simulink model "SPIcontroller"  (R2014b)
settings: Solver=FixedStepDiscrete  StartTime=0.0  StopTime=inf  FixedStep=1  RelTol=1e-3
undefined symbols (not defined in the file): PROD_ID
libraries: hdlsllib x1, simulink x1
settings Model: Creator=bsoheili  LastModifiedBy=dlwalter
settings DataIOCC: SaveOutput=off  SaveTime=off
settings OptimizationCC: BlockReduction=off  ConditionallyExecuteInputs=off  InlineParams=on  UseDivisionForNetSlopeComputation=UseDivisionForReciprocalsOfIntegersOnly  UseFloatMulNetSlope=on  InlineInvariantSignals=on  EnhancedBackFolding=on  EfficientFloat2IntCast=on  OptimizeModelRefInitCode=on  LifeSpan=1
settings DebuggingCC: AlgebraicLoopMsg=error  InheritedTsInSrcMsg=none  StrictBusMsg=ErrorOnBusTreatedAsVector  NonBusSignalsTreatedAsBus=error
settings HardwareCC: ProdHWDeviceType=ASIC/FPGA->ASIC/FPGA  ProdEqTarget=off
settings RTWCC: SystemTargetFile=ert.tlc  TemplateMakefile=ert_default_tmf  Description=Embedded Coder  GenerateReport=on  ProcessScript=ert_make_rtw_hook  IncludeHyperlinkInReport=on  LaunchReport=on  GenerateTraceInfo=on  GenerateTraceReport=on  GenerateTraceReportSl=on  GenerateTraceReportSf=on  GenerateTraceReportEml=on  GenerateCodeMetricsReport=on
settings CodeAppCC: IgnoreCustomStorageClasses=off
settings ERTTargetCC: GenerateSampleERTMain=on  CombineSignalStateStructs=on  SuppressErrorStatus=on  InlinedParameterPlacement=NonHierarchical  ERTCustomFileTemplate=example_file_process.tlc

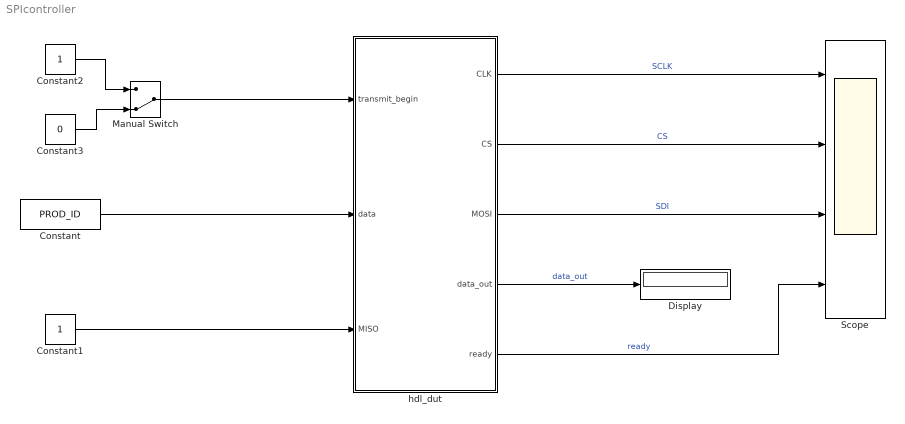
== system SPIcontroller ==
  Constant : Constant  Value=PROD_ID  OutDataTypeStr=fixdt(0,16,0)  SampleTime=-1
  Constant1 : Constant  OutDataTypeStr=boolean  SampleTime=-1
  Constant2 : Constant  OutDataTypeStr=boolean  SampleTime=-1
  Constant3 : Constant  Value=0  OutDataTypeStr=boolean  SampleTime=-1
  Display : Display
  Manual Switch : ManualSwitch  CurrentSetting=0
  Scope : Scope  NumInputPorts=4
      settings: YMin=-2~-2~-2~-5  YMax=2~2~2~5
  hdl_dut : Subsystem  TreatAsAtomicUnit=on  mask{message_length=16, clk_freq=1e6, cs_to_clk_edge=40, stall_time=2}
      mask DialogControl Control2 Prompt: SPI Controller Parameters
      mask DialogControl Control6 Prompt: Message Length (bits)
      mask DialogControl Control3 Prompt: Clock Frequency
      mask DialogControl Control4 Prompt: Chip Select to Clock edge Time (ns)
      mask DialogControl Control5 Prompt: Stall Time (us)
  wires:
  Constant/1 -> hdl_dut/2(data)
  Constant2/1 -> Manual Switch/1
  Constant3/1 -> Manual Switch/2
  Manual Switch/1 -> hdl_dut/1(transmit_begin)
  Constant1/1 -> hdl_dut/3(MISO)
  hdl_dut/1(CLK) -> Scope/1  "SCLK"
  hdl_dut/2(CS) -> Scope/2  "CS"
  hdl_dut/3(MOSI) -> Scope/3  "SDI"
  hdl_dut/4(data_out) -> Display/1  "data_out"
  hdl_dut/5(ready) -> Scope/4  "ready"

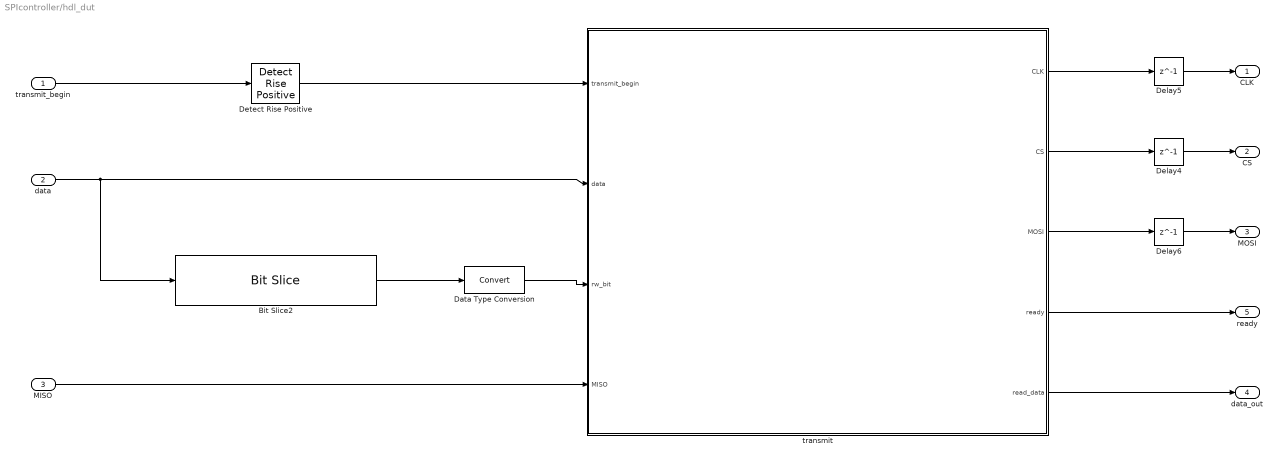
== system SPIcontroller/hdl_dut ==
  transmit_begin : Inport
  data : Inport  Port=2
  MISO : Inport  Port=3
  Bit Slice2 : hdlsllib/HDL Operations/Bit Slice  lidx=message_length-1  ridx=message_length-1
  Data Type Conversion : DataTypeConversion
  Delay4 : Delay  DelayLength=1  InitialCondition=1
  Delay5 : Delay  DelayLength=1  InitialCondition=1
  Delay6 : Delay  DelayLength=1  InitialCondition=0
  Detect Rise Positive : simulink/Logic and Bit Operations/Detect Rise Positive  vinit=0  InputProcessing=Inherited  OutDataTypeStr=boolean
  transmit : Stateflow chart  TreatAsAtomicUnit=on
  CLK : Outport
  CS : Outport  Port=2
  MOSI : Outport  Port=3
  data_out : Outport  Port=4
  ready : Outport  Port=5
  wires:
  data/1 -> Bit Slice2/1, transmit/2(data)
  Delay4/1 -> CS/1
  Delay5/1 -> CLK/1
  Delay6/1 -> MOSI/1
  Bit Slice2/1 -> Data Type Conversion/1
  transmit_begin/1 -> Detect Rise Positive/1
  Data Type Conversion/1 -> transmit/3(rw_bit)
  MISO/1 -> transmit/4(MISO)
  Detect Rise Positive/1 -> transmit/1(transmit_begin)
  transmit/2(CS) -> Delay4/1
  transmit/1(CLK) -> Delay5/1
  transmit/3(MOSI) -> Delay6/1
  transmit/5(read_data) -> data_out/1
  transmit/4(ready) -> ready/1

== stateflow chart SPIcontroller/hdl_dut/transmit ==
  settings: executeAtInitialization=1
  state IDLE
  state BEGIN
  state CHIPSELECT
  state WRITE
    state CLOCK_BEGIN
    state CLOCK_HIGH
    state CLOCK_LOW
    state CLOCK_END
    (default) -> CLOCK_BEGIN
    CLOCK_BEGIN -> CLOCK_LOW : {CLK = false;
        | bit_count = 0;}
    CLOCK_LOW -> CLOCK_HIGH [order 1] : [count == clk_wait]
        | {CLK = 1; count = 0;bit_count ++;
        | MOSI = sdi_gen(data, bit_count);}
    CLOCK_HIGH -> CLOCK_HIGH [order 3] : {count++;}
    CLOCK_LOW -> CLOCK_LOW [order 2] : {count++;}
    CLOCK_HIGH -> CLOCK_LOW [order 1] : [count == clk_wait]
        | {CLK = 0; count = 0;}
    CLOCK_HIGH -> CLOCK_END [order 2] : [bit_count == message_length]
        | {count = 0; transmit_flag = 0; MOSI = 0;}
  state READ
    state CLOCK_BEGIN1
    state BEGIN_READ
    state CLOCK_HIGH1
    state CLOCK_LOW1
    state CS_LOW
    state CLOCK_BEGIN2
    state CLOCK_END1
    state STALL1
    state CLOCK_HIGH2
    state CLOCK_LOW2
    state CLOCK_END2
    (default) -> CLOCK_BEGIN1
    CLOCK_BEGIN1 -> CLOCK_LOW1 : {CLK = false;
        | bit_count = 0;}
    STALL1 -> BEGIN_READ [order 1] : [count == stall_wait]
        | {count = 0;}
    BEGIN_READ -> BEGIN_READ [order 2] : {count++;}
    CLOCK_LOW1 -> CLOCK_HIGH1 [order 1] : [count == clk_wait]
        | {CLK = 1; count = 0;bit_count ++;
        | MOSI = sdi_gen(data, bit_count);}
    CLOCK_HIGH1 -> CLOCK_HIGH1 [order 3] : {count++;}
    CLOCK_LOW1 -> CLOCK_LOW1 [order 2] : {count++;}
    BEGIN_READ -> CS_LOW [order 1] : [count == 10]{CS = 0;count = 0;}
    CLOCK_HIGH1 -> CLOCK_LOW1 [order 1] : [count == clk_wait]
        | {CLK = 0; count = 0;}
    CLOCK_HIGH1 -> CLOCK_END1 [order 2] : [bit_count == message_length]
        | {count = 0; MOSI = 0;}
    CS_LOW -> CS_LOW [order 2] : {count++;}
    CS_LOW -> CLOCK_BEGIN2 [order 1] : [count == cs_wait]
        | {count = 0;}
    CLOCK_END1 -> CLOCK_END1 [order 2] : {count++;}
    STALL1 -> STALL1 [order 2] : {count++;}
    CLOCK_END1 -> STALL1 [order 1] : [count == cs_wait]
        | {count = 0; CS = 1;}
    CLOCK_BEGIN2 -> CLOCK_LOW2 : {CLK = false;
        | bit_count = 0; read_bit = MISO; read_temp = 0;}
    CLOCK_LOW2 -> CLOCK_HIGH2 [order 1] : [count == clk_wait]
        | {CLK = 1; count = 0;bit_count ++;
        | read_temp = read_temp<<1;
        | read_temp = read_temp|read_bit;}
    CLOCK_HIGH2 -> CLOCK_HIGH2 [order 3] : {count++;}
    CLOCK_LOW2 -> CLOCK_LOW2 [order 2] : {count++;}
    CLOCK_HIGH2 -> CLOCK_LOW2 [order 1] : [count == clk_wait]
        | {CLK = 0; count = 0;}
    CLOCK_HIGH2 -> CLOCK_END2 [order 2] : [bit_count == message_length]
        | {count = 0; MOSI = 0; read_data = read_temp; transmit_flag = 0;}
  state END_TRANS
  state STALL
  (default) -> IDLE : {ready = 1;}
  STALL -> IDLE [order 1] : [count == stall_wait]
      | {ready = 1;}
  IDLE -> BEGIN : [transmit_begin == 1]
      | {ready = 0;transmit_flag = 1;count = 0;CS = 1; CLK = 1;}
  BEGIN -> CHIPSELECT : {CS = 0;}
  CHIPSELECT -> CHIPSELECT [order 2] : {count++;}
  CHIPSELECT -> (junction 137) [order 1] : [count == cs_wait]{count = 0;}
  (junction 137) -> READ [order 1] : [rw_bit == 0]
  (junction 137) -> WRITE [order 2] : [rw_bit == 1]
  WRITE -> END_TRANS : [transmit_flag == 0]
  READ -> END_TRANS : [transmit_flag == 0]
  END_TRANS -> END_TRANS [order 2] : {count++;}
  END_TRANS -> STALL [order 1] : [count == cs_wait]{count = 0; CS = 1;}
  STALL -> STALL [order 2] : {count++;}
  data: word function_input fixdt(0,16,0); cnt function_input fixdt(0,5,0); ser_data function_output boolean; CLK output boolean =true; CS output boolean =true; transmit_begin input boolean; data input fixdt(0,message_length,0); clk_wait local fixdt(0,16,0) =floor(12.5e6/clk_freq); clk_freq parameter fixdt(0,32,0); stall_time parameter fixdt(0,16,0); cs_to_clk_edge parameter fixdt(0,16,0); stall_wait local fixdt(0,16,0) =ceil(stall_time/.04); cs_wait local fixdt(0,16,0) =ceil(cs_to_clk_edge/40); rw_bit input boolean; message_length parameter fixdt(0,16,0); count local fixdt(0,16,0); bit_count local fixdt(0,16,0); MOSI output boolean; MISO input boolean; ready output boolean =1; transmit_flag local boolean; read_bit local fixdt(0,message_length,0); read_temp local fixdt(0,message_length,0); read_data output fixdt(0,message_length,0)
  function ser_data = sdi_gen(word,cnt):
    | function ser_data = sdi_gen(word,cnt)
    | 
    | 
    | persistent ser_data_int;
    | if isempty(ser_data_int)
    |     ser_data_int = false;
    | end
    | 
    | 
    | if cnt == fi(1,0,5,0)
    |     ser_data_int = logical(bitget(word, 16));
    | elseif cnt == fi(2,0,5,0)
    |     ser_data_int = logical(bitget(word, 15));
    | elseif cnt == fi(3,0,5,0)
    |     ser_data_int = logical(bitget(word, 14));
    | elseif cnt == fi(4,0,5,0)
    |     ser_data_int = logical(bitget(word, 13));
    | elseif cnt == fi(5,0,5,0)
    |     ser_data_int = logical(bitget(word, 12));
    | elseif cnt == fi(6,0,5,0)
    |     ser_data_int = logical(bitget(word, 11));
    | elseif cnt == fi(7,0,5,0)
    |     ser_data_int = logical(bitget(word, 10));
    | elseif cnt == fi(8,0,5,0)
    |     ser_data_int = logical(bitget(word, 9));
    | elseif cnt == fi(9,0,5,0)
    |     ser_data_int = logical(bitget(word, 8));
    | elseif cnt == fi(10,0,5,0)
    |     ser_data_int = logical(bitget(word, 7));
    | elseif cnt == fi(11,0,5,0)
    |     ser_data_int = logical(bitget(word, 6));
    | elseif cnt == fi(12,0,5,0)
    |     ser_data_int = logical(bitget(word, 5));
    | elseif cnt == fi(13,0,5,0)
    |     ser_data_int = logical(bitget(word, 4));
    | elseif cnt == fi(14,0,5,0)
    |     ser_data_int = logical(bitget(word, 3));
    | elseif cnt == fi(15,0,5,0)
    |     ser_data_int = logical(bitget(word, 2));
    | elseif cnt == fi(16,0,5,0)
    |     ser_data_int = logical(bitget(word, 1));    
    | else
    |     ser_data_int = true;
    | end
    | 
    | ser_data = ser_data_int;
